simulink model "question3"  (R2020b)
settings: Solver=VariableStepAuto  StartTime=0.0  StopTime=10.0  MaxStep=0.001  RelTol=1e-3
settings Model: Creator=Ravi  LastModifiedBy=Ravi

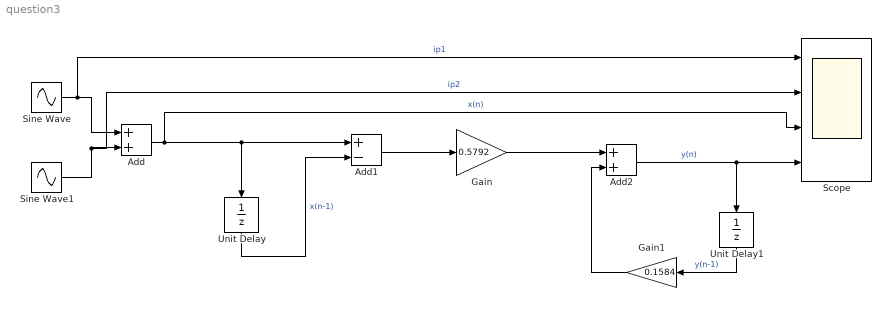
== system question3 ==
  Add : Sum
  Add1 : Sum  Inputs=+-
  Add2 : Sum
  Gain : Gain  Gain=0.5792
  Gain1 : Gain  Gain=0.1584
  Scope : Scope  NumInputPorts=4
  Sine Wave : Sin  SampleTime=0
  Sine Wave1 : Sin  Amplitude=0.5  Frequency=50  SampleTime=0
  Unit Delay : UnitDelay  SampleTime=-1  HasFrameUpgradeWarning=on
  Unit Delay1 : UnitDelay  SampleTime=-1  HasFrameUpgradeWarning=on
  wires:
  Sine Wave/1 -> Scope/1, Add/1  "ip1"
  Sine Wave1/1 -> Scope/2, Add/2  "ip2"
  Add/1 -> Scope/3, Unit Delay/1, Add1/1  "x(n)"
  Unit Delay/1 -> Add1/2  "x(n-1)"
  Add1/1 -> Gain/1
  Gain/1 -> Add2/1
  Add2/1 -> Scope/4, Unit Delay1/1  "y(n)"
  Unit Delay1/1 -> Gain1/1  "y(n-1)"
  Gain1/1 -> Add2/2
